simulink model "W08_P1"  (R2024b)
settings: Solver=ode4  StartTime=0  StopTime=T_final  FixedStep=h  RelTol=1e-3
undefined symbols (not defined in the file or in its folder): beta_c, h, k_neg, k_pos, mp, R_arrive, rp, T_hold, T_max, T_min, V_c, WP_E, WP_N, x0, y_pont
settings Model: Creator=admin  LastModifiedBy=admin
settings DataIOCC: ReturnWorkspaceOutputs=off

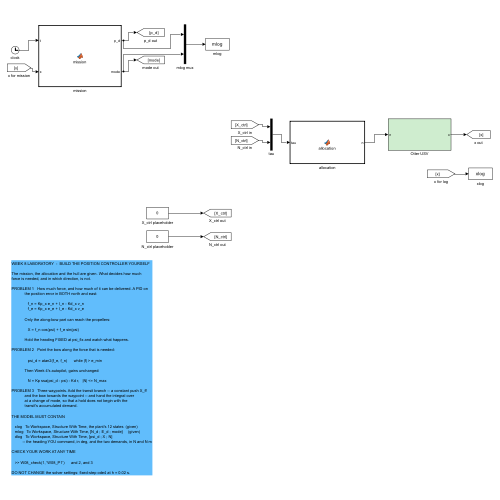
[thumbnail: Simulink's stored preview of the top-level diagram]
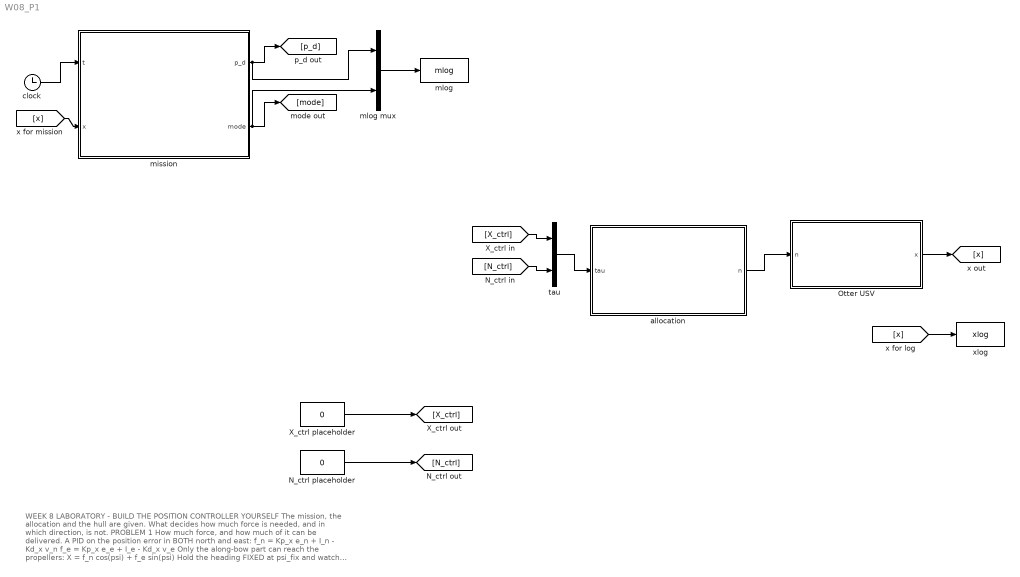
== system W08_P1 ==
  note: WEEK 8 LABORATORY  -  BUILD THE POSITION CONTROLLER YOURSELF
      |
      | The mission, the allocation and the hull are given. What decides how much
      | force is needed, and in which direction, is not.
      |
      | PROBLEM 1   How much force, and how much of it can be delivered. A PID on
      |             the position error in BOTH north and east:
      |
      |                f_n = Kp_x e_n + I_n - Kd_x v_n
      |                f_e = Kp_x e_e + I_e - Kd_x v_e
      |
      |             Only the along-bow part can reach the propellers:
      |
      |                X = f_n cos(psi) + f_e sin(psi)
      |
      |             Hold the heading FIXED at psi_fix and watch what happens.
      |
      | PROBLEM 2   Point the bow along the force that is needed:
      |
      |                psi_d = atan2(f_e, f_n)      while |f| > e_min
      |
      |             Then Week 4's autopilot, gains unchanged:
      |
      |                N = Kp ssa(psi_d - psi) - Kd r,   |N| <= N_max
      |
      | PROBLEM 3   Three waypoints. Add the transit branch -- a constant push X_ff
      |             and the bow towards the waypoint -- and hand the integral over
      |             at a change of mode, so that a hold does not begin with the
      |             transit's accumulated demand.
      |
      | THE MODEL MUST CONTAIN
      |
      |    xlog   To Workspace, Structure With Time, the plant's 12 states  (given)
      |    mlog   To Workspace, Structure With Time, [N_d ; E_d ; mode]     (given)
      |    dlog   To Workspace, Structure With Time, [psi_d ; X ; N]
      |           -- the heading YOU command, in deg, and the two demands, in N and N m
      |
      | CHECK YOUR WORK AT ANY TIME
      |
      |    >> W08_check(1, 'W08_P1')      and 2, and 3
      |
      | DO NOT CHANGE the solver settings: fixed-step ode4 at h = 0.02 s.
  N_ctrl placeholder : Constant  Value=0
  Otter USV : Subsystem
  X_ctrl placeholder : Constant  Value=0
  allocation : MATLAB Function  TreatAsAtomicUnit=on
  clock : Clock
  mission : MATLAB Function  TreatAsAtomicUnit=on
  mlog : ToWorkspace  VariableName=mlog  SaveFormat=Structure With Time  SampleTime=-1
  mlog mux : Mux  Inputs=2
  tau : Mux  Inputs=2
  xlog : ToWorkspace  VariableName=xlog  SaveFormat=Structure With Time  SampleTime=-1
  wires:
  clock/1 -> mission/1(t)
  [x] -> mission/2(x)
  mission/1(p_d) -> [p_d], mlog mux/1
  mission/2(mode) -> [mode], mlog mux/2
  mlog mux/1 -> mlog/1
  [X_ctrl] -> tau/1
  [N_ctrl] -> tau/2
  tau/1 -> allocation/1(tau)
  allocation/1(n) -> Otter USV/1(n)
  Otter USV/1(x) -> [x]
  [x] -> xlog/1
  X_ctrl placeholder/1 -> [X_ctrl]
  N_ctrl placeholder/1 -> [N_ctrl]

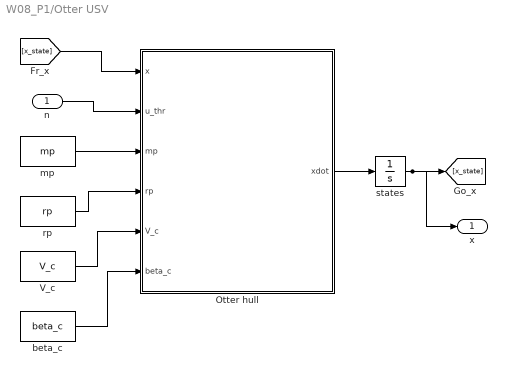
== system W08_P1/Otter USV ==
  n : Inport
  Otter hull : MATLAB Function  TreatAsAtomicUnit=on
  V_c : Constant  Value=V_c
  beta_c : Constant  Value=beta_c
  mp : Constant  Value=mp
  rp : Constant  Value=rp
  states : Integrator  InitialCondition=x0
  x : Outport
  wires:
  [x_state] -> Otter hull/1(x)
  rp/1 -> Otter hull/4(rp)
  n/1 -> Otter hull/2(u_thr)
  beta_c/1 -> Otter hull/6(beta_c)
  mp/1 -> Otter hull/3(mp)
  V_c/1 -> Otter hull/5(V_c)
  Otter hull/1(xdot) -> states/1
  states/1 -> [x_state], x/1

== matlab function W08_P1/allocation ==
  data: tau input; n output double size=[2 1]; y_pont parameter; k_pos parameter; k_neg parameter; T_max parameter; T_min parameter
function n = allocation(tau, y_pont, k_pos, k_neg, T_max, T_min)
%#codegen
%  6주차의 배분 그대로 / the allocation of Week 6, unchanged
T1 = tau(1)/2 + tau(2)/(2*y_pont);
T2 = tau(1)/2 - tau(2)/(2*y_pont);
s = 1;
if T1 > T_max, s = min(s, T_max/T1); end
if T2 > T_max, s = min(s, T_max/T2); end
if T1 < T_min, s = min(s, T_min/T1); end
if T2 < T_min, s = min(s, T_min/T2); end
T1 = s*T1;  T2 = s*T2;
k1 = k_pos;  if T1 < 0, k1 = k_neg; end
k2 = k_pos;  if T2 < 0, k2 = k_neg; end
n = [sign(T1)*sqrt(abs(T1)/k1); sign(T2)*sqrt(abs(T2)/k2)];

== matlab function W08_P1/mission ==
  settings: updateMethod=DISCRETE  sampleTime=h
  data: t input; p_d output double size=[2 1]; x input; mode output; WP_N parameter; WP_E parameter; R_arrive parameter; T_hold parameter; h parameter
function [p_d, mode] = mission(t, x, WP_N, WP_E, R_arrive, T_hold, h)
%#codegen
%MISSION  8주차 §8-5 의 상태기계. 규칙은 둘뿐이다.
%         The state machine of Week 8 §8-5: two rules only.
%
%    이동 중이고 목표에 R_arrive 안으로 들어오면  -> 유지, 시계를 0 으로
%    유지 중이고 T_hold 가 지나면                -> 다음 지점, 이동으로
%
%    in transit and inside R_arrive  -> hold, and reset the clock
%    in hold and T_hold has passed   -> the next waypoint, and transit
%
%  웨이포인트가 하나뿐이면 배는 처음부터 유지 모드에 있고 거기 머문다 —
%  1·2번 문제가 원하는 것이 그것이다.
%  With a single waypoint the vessel starts in hold and stays there, which is
%  what Problems 1 and 2 want.
persistent k mode_ held
if isempty(k), k = 1; mode_ = 1; held = 0; end
d = hypot(WP_N(k) - x(7), WP_E(k) - x(8));
if mode_ == 1 && d < R_arrive
    mode_ = 2;  held = 0;
elseif mode_ == 2
    held = held + h;
    if held >= T_hold
        if k < numel(WP_N), k = k + 1;  mode_ = 1;  else, mode_ = 3; end
    end
end
p_d  = [WP_N(k); WP_E(k)];
mode = mode_;

== matlab function W08_P1/Otter USV/Otter hull ==
  data: x input; xdot output double size=[12 1]; u_thr input; mp input; rp input; V_c input; beta_c input
function xdot = otter_hull(x, u_thr, mp, rp, V_c, beta_c)
% Fossen's otter.m, called unchanged from Tools/MSS/VESSELS.
%
%   x       12 states, fed back from the integrator
%   u_thr   propeller shaft speeds [rad/s]
%
% otter.m is not written for code generation, so the call is extrinsic and
% xdot has to be pre-sized for Simulink to know the output width.
coder.extrinsic('otter');

xdot = zeros(12,1);
xdot = otter(x, u_thr, mp, rp, V_c, beta_c);
end
